simulink model "Ex02"  (R2021b)
settings: Solver=VariableStepAuto  StartTime=0.0  StopTime=10.0  RelTol=1e-3
settings Model: Creator=carlo  LastModifiedBy=carlo
settings SolverCC: AlgebraicLoopSolver=TrustRegion
settings DebuggingCC: SFMachineParentedDataDiag=warning

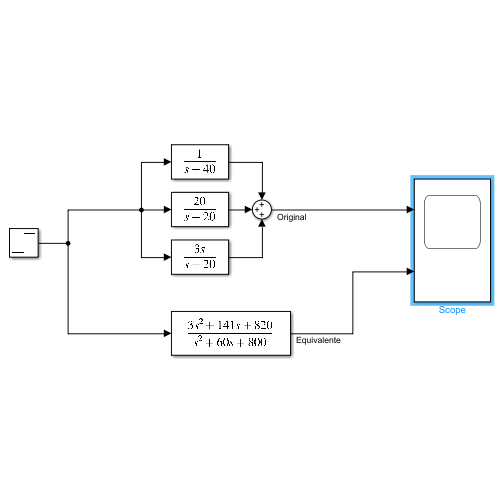
[thumbnail: Simulink's stored preview of the top-level diagram]
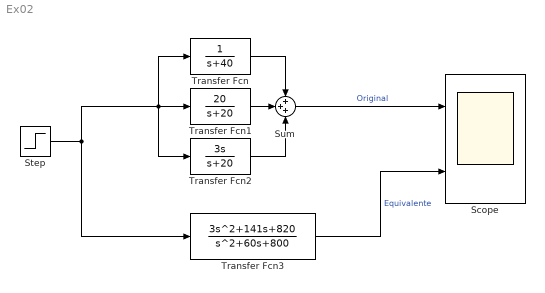
== system Ex02 ==
  Scope : Scope  NumInputPorts=2
  Step : Step  SampleTime=0
  Sum : Sum  Inputs=+++
  Transfer Fcn : TransferFcn  Numerator=1  Denominator=[1 40]
  Transfer Fcn1 : TransferFcn  Numerator=20  Denominator=[1 20]
  Transfer Fcn2 : TransferFcn  Numerator=[3 0]  Denominator=[1 20]
  Transfer Fcn3 : TransferFcn  Numerator=[3 141 820]  Denominator=[1 60 800]
  wires:
  Transfer Fcn/1 -> Sum/1
  Transfer Fcn1/1 -> Sum/2
  Sum/1 -> Scope/1  "Original"
  Step/1 -> Transfer Fcn3/1, Transfer Fcn/1, Transfer Fcn2/1, Transfer Fcn1/1
  Transfer Fcn2/1 -> Sum/3
  Transfer Fcn3/1 -> Scope/2  "Equivalente"
